simulink model "Main"  (R2020b)
settings: Solver=VariableStepAuto  StartTime=0.0  StopTime=inf  RelTol=1e-3
libraries: TcSimInterface x1
(part 2 of 2)

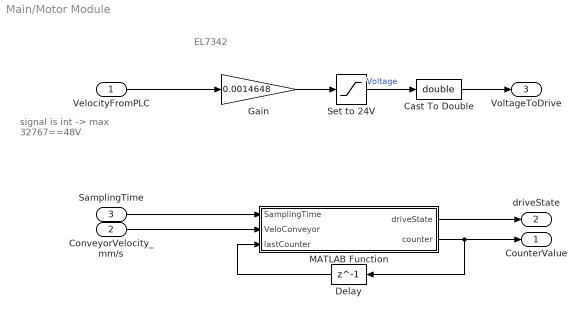
== system Main/Motor Module ==
  note: signal is int ->
      | max 32767==48V
  note: EL7342
  VelocityFromPLC : Inport
  ConveyorVelocity_mm/s : Inport  Port=2
  SamplingTime : Inport  Port=3
  Cast To Double : DataTypeConversion  OutDataTypeStr=double
  Delay : Delay  DelayLength=1
  Gain : Gain  Gain=0.0014648
  MATLAB Function : MATLAB Function  TreatAsAtomicUnit=on
  Set to 24V : Saturate  UpperLimit=24  LowerLimit=-24
  CounterValue : Outport
  driveState : Outport  Port=2
  VoltageToDrive : Outport  Port=3
  wires:
  Gain/1 -> Set to 24V/1
  Cast To Double/1 -> VoltageToDrive/1
  MATLAB Function/2(counter) -> Delay/1, CounterValue/1
  ConveyorVelocity_mm/s/1 -> MATLAB Function/2(VeloConveyor)
  MATLAB Function/1(driveState) -> driveState/1
  Set to 24V/1 -> Cast To Double/1  "Voltage"
  Delay/1 -> MATLAB Function/3(lastCounter)
  SamplingTime/1 -> MATLAB Function/1(SamplingTime)
  VelocityFromPLC/1 -> Gain/1

== matlab function Main/Motor Module/MATLAB Function ==
  data: driveState output; SamplingTime input; VeloConveyor input; counter output; lastCounter input
function [driveState,counter] = fcn(SamplingTime, VeloConveyor, lastCounter)
%%
%    VeloConveyor in mm/s
%    SamplingTime in s
%    lastCounter 1count = 0.0001mm

%%
driveState = uint8(0);
driveState = bitset(driveState,1,1);    % Ready to enable
driveState = bitset(driveState,2,1);    % Ready 
if (VeloConveyor > 0)
    driveState = bitset(driveState,5,1);    % Moving Positive
elseif (VeloConveyor < 0)
    driveState = bitset(driveState,6,1);    % Moving Negative
end

diff = VeloConveyor*SamplingTime*10000;
if (lastCounter+diff >= 65535)
    counter = lastCounter+diff -65535;
else
    counter = lastCounter + VeloConveyor*SamplingTime*10000;
end

end

== matlab function Main/Encode ==
  data: counterValue input; modelToPlc output; driveState input
function modelToPlc = EncodePlcMessage(counterValue, driveState)
    modelToPlc = uint32(0);
    modelToPlc = bitor(modelToPlc, uint32(driveState));
    modelToPlc = bitshift(modelToPlc,16);
    
    modelToPlc = bitor(modelToPlc, uint32(counterValue));
    
    %modelToPlc = bitand(modelToPlc, bitshift(driveState,16));
    %modelToPlc = bitand(modelToPlc, counterValue);

end

== matlab function Main/Decode ==
  data: PlcToModel input; velocity output
function velocity  = DecodePlcMessage(PlcToModel)


velocity = bitand(PlcToModel, uint32(0xffff));

end
